simulink model "example_use_sfunctions_2016bb"  (R2016b)
settings: Solver=FixedStepAuto  StartTime=0.0  StopTime=10.0  FixedStep=0.01  RelTol=1e-3
libraries: dspnetwork x2, etargetslib x1, aerolibanimutils x1
settings Model: Creator=Admin  LastModifiedBy=luminghua

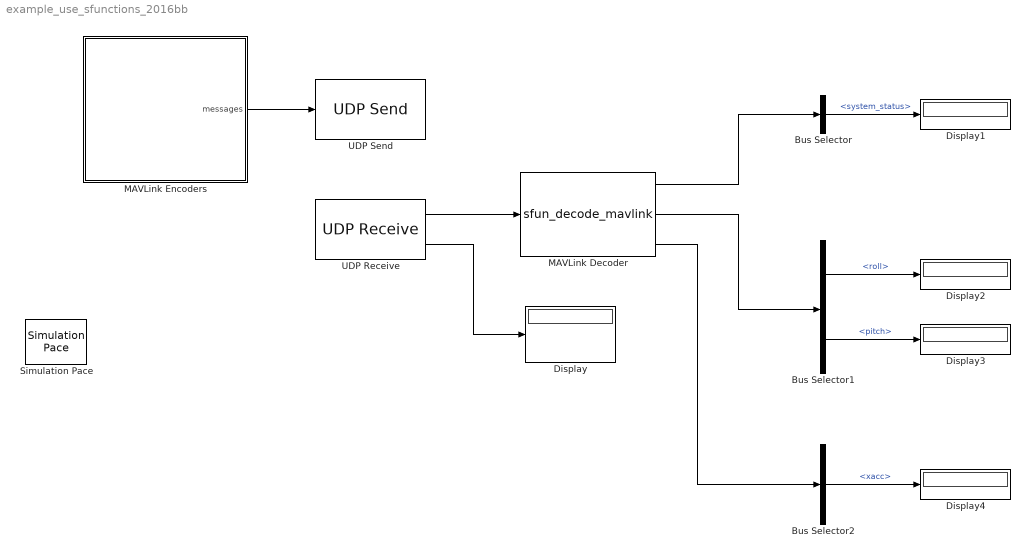
== system example_use_sfunctions_2016bb ==
  Bus Selector : BusSelector  OutputSignals=system_status
  Bus Selector1 : BusSelector  OutputSignals=roll,pitch
  Bus Selector2 : BusSelector  OutputSignals=xacc
  Display{,1..4} (5 alike) : Display
  MAVLink Decoder : S-Function  FunctionName=sfun_decode_mavlink  SFunctionDeploymentMode=off  EnableBusSupport=off
  MAVLink Encoders : Subsystem
  Simulation Pace : aerolibanimutils/Simulation Pace  SimulationPace=1  SleepMode=MATLAB Thread  OutputPaceError=off  SampleTime=0.01
  UDP Receive : dspnetwork/UDP Receive  localURL='0.0.0.0'  localPort=14550  remoteURL='0.0.0.0'  remotePort=-1  recvBufferSize=8192  dims=263  signalDatatype=uint8  isVarSize=off  showBlockingTime=on  blockingTime=0  sampletime=0.01  blockPlatform=HOST
  UDP Send : dspnetwork/UDP Send  remoteURL='255.255.255.255'  remotePort=25000  localURL='0.0.0.0'  localPortSource=Automatically determine  localPort=-1  sampletime=-1  blockPlatform=HOST  separateLengthPort=0
  wires:
  MAVLink Encoders/1(messages) -> UDP Send/1
  UDP Receive/1 -> MAVLink Decoder/1
  UDP Receive/2 -> Display/1
  MAVLink Decoder/1 -> Bus Selector/1
  MAVLink Decoder/2 -> Bus Selector1/1
  Bus Selector/1 -> Display1/1  "<system_status>"
  Bus Selector1/1 -> Display2/1  "<roll>"
  Bus Selector1/2 -> Display3/1  "<pitch>"
  MAVLink Decoder/3 -> Bus Selector2/1
  Bus Selector2/1 -> Display4/1  "<xacc>"

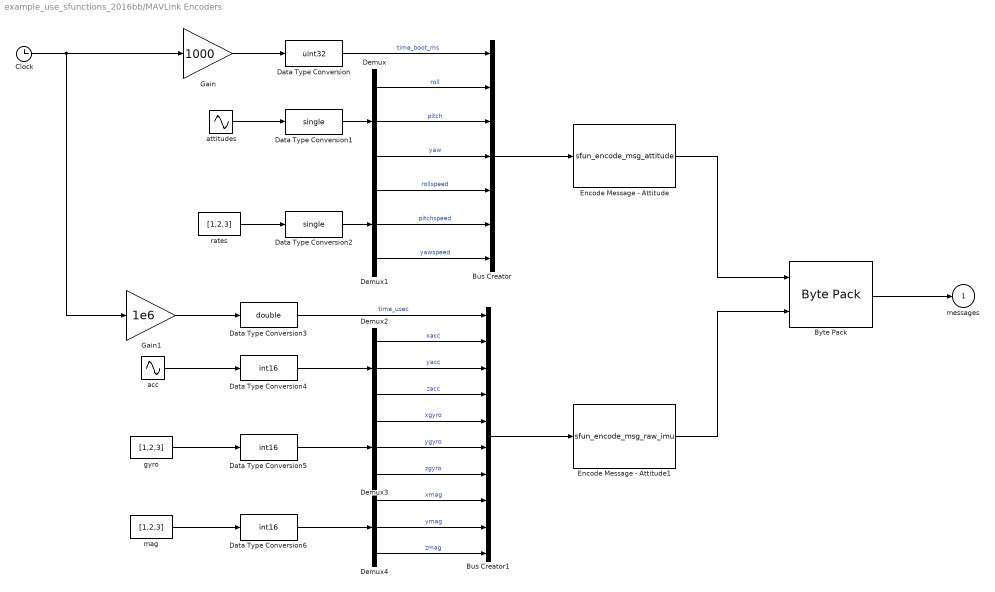
== system example_use_sfunctions_2016bb/MAVLink Encoders ==
  Bus Creator : BusCreator  Inputs=7  OutDataTypeStr=Bus: mavlink_attitude_t
  Bus Creator1 : BusCreator  Inputs=10  OutDataTypeStr=Bus: mavlink_raw_imu_t
  Byte Pack : etargetslib/Byte Pack  datatypes={'uint8','uint8'}  byteAlign=1
  Clock : Clock
  Data Type Conversion : DataTypeConversion  OutDataTypeStr=uint32
  Data Type Conversion1 : DataTypeConversion  OutDataTypeStr=single
  Data Type Conversion2 : DataTypeConversion  OutDataTypeStr=single
  Data Type Conversion3 : DataTypeConversion  OutDataTypeStr=double
  Data Type Conversion4 : DataTypeConversion  OutDataTypeStr=int16
  Data Type Conversion5 : DataTypeConversion  OutDataTypeStr=int16
  Data Type Conversion6 : DataTypeConversion  OutDataTypeStr=int16
  Demux{,1..4} (5 alike) : Demux  Outputs=3
  Encode Message - Attitude : S-Function  FunctionName=sfun_encode_msg_attitude  SFunctionDeploymentMode=off  EnableBusSupport=off
  Encode Message - Attitude1 : S-Function  FunctionName=sfun_encode_msg_raw_imu  SFunctionDeploymentMode=off  EnableBusSupport=off
  Gain : Gain  Gain=1000
  Gain1 : Gain  Gain=1e6
  acc : Sin  Amplitude=[1000, 1000, 1000]  Phase=[0, pi/2, 0]  SampleTime=0
  attitudes : Sin  Amplitude=[45, 45, 45]  Phase=[0, pi/2, 0]  SampleTime=0
  gyro : Constant  Value=[1,2,3]
  mag : Constant  Value=[1,2,3]
  rates : Constant  Value=[1,2,3]
  messages : Outport
  wires:
  Gain/1 -> Data Type Conversion/1
  Demux1/3 -> Bus Creator/7  "yawspeed"
  Data Type Conversion2/1 -> Demux1/1
  Demux1/2 -> Bus Creator/6  "pitchspeed"
  Data Type Conversion1/1 -> Demux/1
  Demux/3 -> Bus Creator/4  "yaw"
  attitudes/1 -> Data Type Conversion1/1
  Bus Creator/1 -> Encode Message - Attitude/1
  Demux1/1 -> Bus Creator/5  "rollspeed"
  rates/1 -> Data Type Conversion2/1
  Demux/2 -> Bus Creator/3  "pitch"
  Demux/1 -> Bus Creator/2  "roll"
  Data Type Conversion/1 -> Bus Creator/1  "time_boot_ms"
  Clock/1 -> Gain1/1, Gain/1
  Bus Creator1/1 -> Encode Message - Attitude1/1
  Byte Pack/1 -> messages/1
  Encode Message - Attitude/1 -> Byte Pack/1
  Encode Message - Attitude1/1 -> Byte Pack/2
  Data Type Conversion3/1 -> Bus Creator1/1  "time_usec"
  Gain1/1 -> Data Type Conversion3/1
  Demux2/1 -> Bus Creator1/2  "xacc"
  Demux2/2 -> Bus Creator1/3  "yacc"
  Demux2/3 -> Bus Creator1/4  "zacc"
  Demux3/1 -> Bus Creator1/5  "xgyro"
  Demux3/2 -> Bus Creator1/6  "ygyro"
  Demux3/3 -> Bus Creator1/7  "zgyro"
  Demux4/1 -> Bus Creator1/8  "xmag"
  Demux4/2 -> Bus Creator1/9  "ymag"
  Demux4/3 -> Bus Creator1/10  "zmag"
  Data Type Conversion6/1 -> Demux4/1
  Data Type Conversion5/1 -> Demux3/1
  Data Type Conversion4/1 -> Demux2/1
  gyro/1 -> Data Type Conversion5/1
  mag/1 -> Data Type Conversion6/1
  acc/1 -> Data Type Conversion4/1
